simulink model "lorentzsimu"  (R2017b)
settings: Solver=ode4  StartTime=0.0  StopTime=10  FixedStep=1e-5  RelTol=1e-3
values from neighbouring files (symbols this model uses):
  beta = 2    [TEA_Ejercicios0_control_barco_sMatlab.m]    (also in lorentz.m = 2.66666666667; lorentzlqr.m = 2.66666666667)
  init1 = 10-i    [lorentz.m]
  init2 = -10-i    [lorentz.m]
  init3 = 10-i    [lorentz.m]
  rho = 28    [lorentz.m]    (also in lorentzlqr.m)
  sigma = 10    [lorentz.m]    (also in lorentzlqr.m)
settings Model: Creator=pablo  LastModifiedBy=pablo

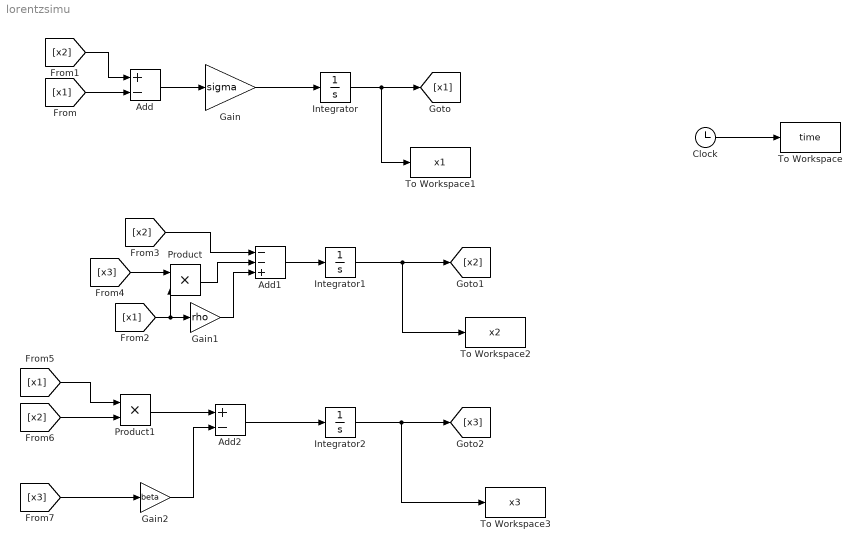
== system lorentzsimu ==
  Add : Sum  Inputs=+-
  Add1 : Sum  Inputs=--+
  Add2 : Sum  Inputs=+-
  Clock : Clock
  Gain : Gain  Gain=sigma
  Gain1 : Gain  Gain=rho
  Gain2 : Gain  Gain=beta
  Integrator : Integrator  InitialCondition=init1
  Integrator1 : Integrator  InitialCondition=init2
  Integrator2 : Integrator  InitialCondition=init3
  Product : Product
  Product1 : Product
  To Workspace : ToWorkspace  VariableName=time  SaveFormat=Timeseries  SampleTime=-1
  To Workspace1 : ToWorkspace  VariableName=x1  SampleTime=-1
  To Workspace2 : ToWorkspace  VariableName=x2  SampleTime=-1
  To Workspace3 : ToWorkspace  VariableName=x3  SampleTime=-1
  wires:
  Gain/1 -> Integrator/1
  Add/1 -> Gain/1
  [x1] -> Add/2
  [x2] -> Add/1
  Integrator/1 -> To Workspace1/1, [x1]
  Add1/1 -> Integrator1/1
  [x1] -> Product/2, Gain1/1
  Gain1/1 -> Add1/3
  [x2] -> Add1/1
  Product/1 -> Add1/2
  [x3] -> Product/1
  Integrator1/1 -> To Workspace2/1, [x2]
  Add2/1 -> Integrator2/1
  Product1/1 -> Add2/1
  [x1] -> Product1/1
  [x2] -> Product1/2
  [x3] -> Gain2/1
  Gain2/1 -> Add2/2
  Integrator2/1 -> To Workspace3/1, [x3]
  Clock/1 -> To Workspace/1
